simulink model "RobotSimulation"  (R2020b)
settings: Solver=ode45  StartTime=0.0  StopTime=2  MaxStep=1e-6  RelTol=1e-3%1e-10
model workspace (MAT data in the model file):
  Mchoice_Planned = Simulink.Parameter
  Mchoice_Planned.Value = 0
  Mchoice_Planned.DataType = 'auto'
  Mchoice_Planned.Dimensions = [1 1]
  robot = robotics.RigidBodyTree
  robot.TreeInternal = robotics.manip.internal.RigidBodyTree
  robot.TreeInternal.NumBodies = 4
  robot.TreeInternal.Base = robotics.manip.internal.RigidBody
  robot.TreeInternal.Base.Index = 0
  robot.TreeInternal.Base.NameInternal = 'base'
  robot.TreeInternal.Base.JointInternal = robotics.Joint
  robot.TreeInternal.Base.JointInternal.Type = 'fixed'
  robot.TreeInternal.Base.JointInternal.VelocityNumber = 0
  robot.TreeInternal.Base.JointInternal.PositionNumber = 0
  robot.TreeInternal.Base.JointInternal.MotionSubspace = [0; 0; 0; 0; 0; 0]
  robot.TreeInternal.Base.JointInternal.NameInternal = 'base_jnt'
  robot.TreeInternal.Base.ParentIndex = -1
  robot.TreeInternal.Base.ChildrenIndices = 1
  robot.TreeInternal.Base.MassInternal = 1
  robot.TreeInternal.Base.CenterOfMassInternal = [0 0 0]
  robot.TreeInternal.Base.InertiaInternal = [1  0  0; 0  1  0; 0  0  1]
  robot.TreeInternal.Base.SpatialInertia = [1  0  0  0  0  0; 0  1  0  0  0  0; 0  0  1  0  0  0; 0  0  0  1  0  0; 0  0  0  0  1  0; 0  0  0  0  0  1]
  robot.TreeInternal.Base.CollisionsInternal = robotics.manip.internal.CollisionSet
  robot.TreeInternal.Base.CollisionsInternal.MaxElements = 0
  robot.TreeInternal.Gravity = [0 0 0]
  robot.TreeInternal.Bodies{1} = robotics.manip.internal.RigidBody
  robot.TreeInternal.Bodies{1}.Index = 1
  robot.TreeInternal.Bodies{1}.NameInternal = 'body1'
  robot.TreeInternal.Bodies{1}.JointInternal = robotics.Joint
  robot.TreeInternal.Bodies{1}.JointInternal.Type = 'revolute'
  robot.TreeInternal.Bodies{1}.JointInternal.VelocityNumber = 1
  robot.TreeInternal.Bodies{1}.JointInternal.PositionNumber = 1
  robot.TreeInternal.Bodies{1}.JointInternal.MotionSubspace = [0; 0; 1; 0; 0; 0]
  robot.TreeInternal.Bodies{1}.JointInternal.InTree = 1
  robot.TreeInternal.Bodies{1}.JointInternal.NameInternal = 'jnt1'
  robot.TreeInternal.Bodies{1}.JointInternal.PositionLimitsInternal = [-3.14159265359 3.14159265359]
  robot.TreeInternal.Bodies{1}.JointInternal.JointAxisInternal = [0 0 1]
  robot.TreeInternal.Bodies{1}.ParentIndex = 0
  robot.TreeInternal.Bodies{1}.ChildrenIndices = [0 1]
  robot.TreeInternal.Bodies{1}.MassInternal = 1
  robot.TreeInternal.Bodies{1}.CenterOfMassInternal = [0 0 0]
  robot.TreeInternal.Bodies{1}.InertiaInternal = [1  0  0; 0  1  0; 0  0  1]
  robot.TreeInternal.Bodies{1}.SpatialInertia = [1  0  0  0  0  0; 0  1  0  0  0  0; 0  0  1  0  0  0; 0  0  0  1  0  0; 0  0  0  0  1  0; 0  0  0  0  0  1]
  robot.TreeInternal.Bodies{1}.CollisionsInternal = robotics.manip.internal.CollisionSet
  robot.TreeInternal.Bodies{1}.CollisionsInternal.MaxElements = 0
  robot.TreeInternal.Bodies{2} = robotics.manip.internal.RigidBody
  robot.TreeInternal.Bodies{2}.Index = 2
  robot.TreeInternal.Bodies{2}.NameInternal = 'body2'
  robot.TreeInternal.Bodies{2}.JointInternal = robotics.Joint
  robot.TreeInternal.Bodies{2}.JointInternal.Type = 'revolute'
  robot.TreeInternal.Bodies{2}.JointInternal.VelocityNumber = 1
  robot.TreeInternal.Bodies{2}.JointInternal.PositionNumber = 1
  robot.TreeInternal.Bodies{2}.JointInternal.MotionSubspace = [0; 0; 1; 0; 0; 0]
  robot.TreeInternal.Bodies{2}.JointInternal.InTree = 1
  robot.TreeInternal.Bodies{2}.JointInternal.JointToParentTransform = [1  0  0  0; 0  1  0  0; 0  0  1  0.2; 0  0  0  1]
  robot.TreeInternal.Bodies{2}.JointInternal.NameInternal = 'jnt2'
  robot.TreeInternal.Bodies{2}.JointInternal.PositionLimitsInternal = [-3.14159265359 3.14159265359]
  robot.TreeInternal.Bodies{2}.JointInternal.JointAxisInternal = [0 0 1]
  robot.TreeInternal.Bodies{2}.ParentIndex = 1
  robot.TreeInternal.Bodies{2}.ChildrenIndices = [0 0 1]
  robot.TreeInternal.Bodies{2}.MassInternal = 1
  robot.TreeInternal.Bodies{2}.CenterOfMassInternal = [0 0 0]
  robot.TreeInternal.Bodies{2}.InertiaInternal = [1  0  0; 0  1  0; 0  0  1]
  robot.TreeInternal.Bodies{2}.SpatialInertia = [1  0  0  0  0  0; 0  1  0  0  0  0; 0  0  1  0  0  0; 0  0  0  1  0  0; 0  0  0  0  1  0; 0  0  0  0  0  1]
  robot.TreeInternal.Bodies{2}.CollisionsInternal = robotics.manip.internal.CollisionSet
  robot.TreeInternal.Bodies{2}.CollisionsInternal.MaxElements = 0
  robot.TreeInternal.Bodies{3} = robotics.manip.internal.RigidBody
  robot.TreeInternal.Bodies{3}.Index = 3
  robot.TreeInternal.Bodies{3}.NameInternal = 'body3'
  robot.TreeInternal.Bodies{3}.JointInternal = robotics.Joint
  robot.TreeInternal.Bodies{3}.JointInternal.Type = 'prismatic'
  robot.TreeInternal.Bodies{3}.JointInternal.VelocityNumber = 1
  robot.TreeInternal.Bodies{3}.JointInternal.PositionNumber = 1
  robot.TreeInternal.Bodies{3}.JointInternal.MotionSubspace = [0; 0; 0; 0; 0; 1]
  robot.TreeInternal.Bodies{3}.JointInternal.InTree = 1
  robot.TreeInternal.Bodies{3}.JointInternal.JointToParentTransform = [1  0  0  0.1; 0  1  0  0; 0  0  1  0; 0  0  0  1]
  robot.TreeInternal.Bodies{3}.JointInternal.NameInternal = 'jnt3'
  robot.TreeInternal.Bodies{3}.JointInternal.PositionLimitsInternal = [-0.5 0.5]
  robot.TreeInternal.Bodies{3}.JointInternal.JointAxisInternal = [0 0 1]
  robot.TreeInternal.Bodies{3}.ParentIndex = 2
  robot.TreeInternal.Bodies{3}.ChildrenIndices = [0 0 0 1]
  robot.TreeInternal.Bodies{3}.MassInternal = 1
  robot.TreeInternal.Bodies{3}.CenterOfMassInternal = [0 0 0]
  robot.TreeInternal.Bodies{3}.InertiaInternal = [1  0  0; 0  1  0; 0  0  1]
  robot.TreeInternal.Bodies{3}.SpatialInertia = [1  0  0  0  0  0; 0  1  0  0  0  0; 0  0  1  0  0  0; 0  0  0  1  0  0; 0  0  0  0  1  0; 0  0  0  0  0  1]
  robot.TreeInternal.Bodies{3}.CollisionsInternal = robotics.manip.internal.CollisionSet
  robot.TreeInternal.Bodies{3}.CollisionsInternal.MaxElements = 0
  robot.TreeInternal.Bodies{4} = robotics.manip.internal.RigidBody
  robot.TreeInternal.Bodies{4}.Index = 4
  robot.TreeInternal.Bodies{4}.NameInternal = 'tool'
  robot.TreeInternal.Bodies{4}.JointInternal = robotics.Joint
  robot.TreeInternal.Bodies{4}.JointInternal.Type = 'fixed'
  robot.TreeInternal.Bodies{4}.JointInternal.VelocityNumber = 0
  robot.TreeInternal.Bodies{4}.JointInternal.PositionNumber = 0
  robot.TreeInternal.Bodies{4}.JointInternal.MotionSubspace = [0; 0; 0; 0; 0; 0]
  robot.TreeInternal.Bodies{4}.JointInternal.InTree = 1
  robot.TreeInternal.Bodies{4}.JointInternal.NameInternal = 'jnt4'
  robot.TreeInternal.Bodies{4}.ParentIndex = 3
  robot.TreeInternal.Bodies{4}.ChildrenIndices = [0 0 0]
  robot.TreeInternal.Bodies{4}.MassInternal = 1
  robot.TreeInternal.Bodies{4}.CenterOfMassInternal = [0 0 0]
  robot.TreeInternal.Bodies{4}.InertiaInternal = [1  0  0; 0  1  0; 0  0  1]
  robot.TreeInternal.Bodies{4}.SpatialInertia = [1  0  0  0  0  0; 0  1  0  0  0  0; 0  0  1  0  0  0; 0  0  0  1  0  0; 0  0  0  0  1  0; 0  0  0  0  0  1]
  robot.TreeInternal.Bodies{4}.CollisionsInternal = robotics.manip.internal.CollisionSet
  robot.TreeInternal.Bodies{4}.CollisionsInternal.MaxElements = 0
  robot.TreeInternal.NumNonFixedBodies = 3
  robot.TreeInternal.PositionNumber = 3
  robot.TreeInternal.VelocityNumber = 3
  robot.TreeInternal.PositionDoFMap = [1  1; 2  2; 3  3; 0  -1]
  robot.TreeInternal.VelocityDoFMap = [1  1; 2  2; 3  3; 0  -1]
  robot.TreeInternal.MaxNumBodies = 4
  robot.TreeInternal.MaxNameLength = 200
  robot.TreeInternal.MaxJointPositionNumber = 7
  robot.TreeInternal.VisualizationInfo = robotics.manip.internal.VisualizationInfo
  robot.TreeInternal.VisualizationInfo.ShowTag = 'DO_NOT_EDIT_qoTUB'
  robot.TreeInternal.DataFormatInternal = 'struct'
settings Model: OrderedModelArguments=off  Creator=alons  LastModifiedBy=alons
settings SolverCC: ConsecutiveZCsStepRelTol=eps%10*128*eps

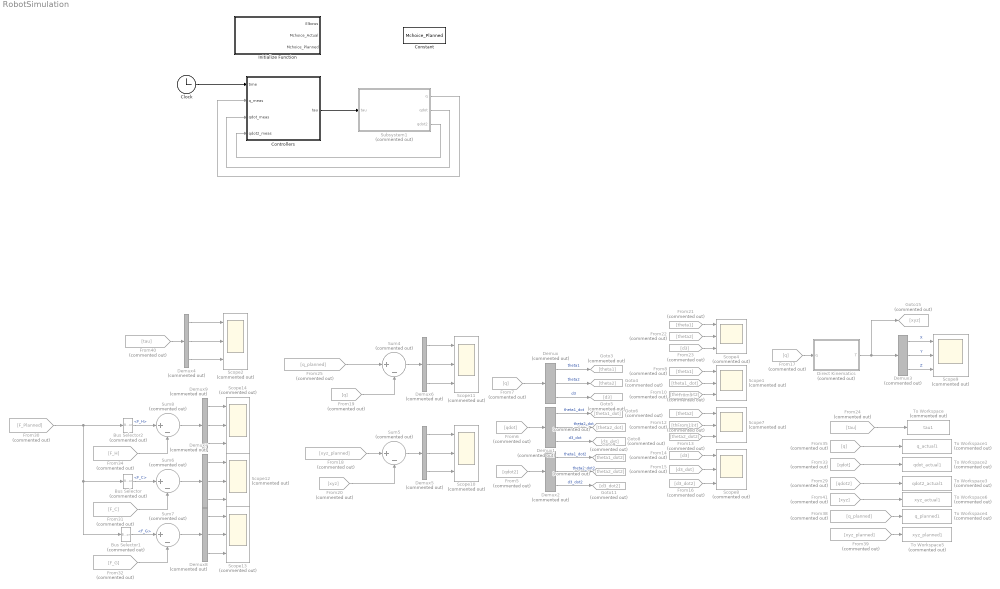
== system RobotSimulation ==
  Bus Selector : BusSelector  Commented=on  OutputSignals=F_C
  Bus Selector1 : BusSelector  Commented=on  OutputSignals=F_G
  Bus Selector2 : BusSelector  Commented=on  OutputSignals=F_H
  Clock : Clock
  Constant : Constant  Value=Mchoice_Planned
  Controllers : Subsystem  TreatAsAtomicUnit=on
      mask Display: disp('Controller')
  Demux{,1..9} (10 alike) : Demux  Commented=on  Outputs=3
  Direct Kinematics : MATLAB Function  Commented=on  TreatAsAtomicUnit=on
  From10 : From  Commented=on  GotoTag=theta1_dot2
  From11 : From  Commented=on  GotoTag=theta2
  From12 : From  Commented=on  GotoTag=theta2_dot
  From13 : From  Commented=on  GotoTag=theta2_dot2
  From14 : From  Commented=on  GotoTag=d3
  From15 : From  Commented=on  GotoTag=d3_dot
  From16 : From  Commented=on  GotoTag=d3_dot2
  From{7,17,19,35} (4 alike) : From  Commented=on  GotoTag=q
  From18 : From  Commented=on  GotoTag=xyz_planned
  From20 : From  Commented=on  GotoTag=xyz
  From21 : From  Commented=on  GotoTag=theta1
  From22 : From  Commented=on  GotoTag=theta2
  From23 : From  Commented=on  GotoTag=d3
  From24 : From  Commented=on  GotoTag=tau
  From25 : From  Commented=on  GotoTag=q_planned
  From29 : From  Commented=on  GotoTag=qdot2
  From30 : From  Commented=on  GotoTag=F_Planned
  From31 : From  Commented=on  GotoTag=F_C
  From32 : From  Commented=on  GotoTag=F_G
  From33 : From  Commented=on  GotoTag=qdot
  From34 : From  Commented=on  GotoTag=F_H
  From38 : From  Commented=on  GotoTag=q_planned
  From39 : From  Commented=on  GotoTag=xyz_planned
  From40 : From  Commented=on  GotoTag=tau
  From41 : From  Commented=on  GotoTag=xyz
  From5 : From  Commented=on  GotoTag=qdot2
  From6 : From  Commented=on  GotoTag=qdot
  From8 : From  Commented=on  GotoTag=theta1
  From9 : From  Commented=on  GotoTag=theta1_dot
  Goto10 : Goto  Commented=on  GotoTag=theta2_dot2
  Goto11 : Goto  Commented=on  GotoTag=d3_dot2
  Goto15 : Goto  Commented=on  GotoTag=xyz
  Goto3 : Goto  Commented=on  GotoTag=theta1
  Goto4 : Goto  Commented=on  GotoTag=theta2
  Goto5 : Goto  Commented=on  GotoTag=d3
  Goto6 : Goto  Commented=on  GotoTag=theta1_dot
  Goto7 : Goto  Commented=on  GotoTag=theta2_dot
  Goto8 : Goto  Commented=on  GotoTag=d3_dot
  Goto9 : Goto  Commented=on  GotoTag=theta1_dot2
  Initialize Function : Subsystem  TreatAsAtomicUnit=on
  Scope{1..2,4,7..14} (11 alike) : Scope  Commented=on  NumInputPorts=3
  Subsystem1 : Subsystem  Commented=on
      mask Display: disp('Plant')
  Sum{4..8} (5 alike) : Sum  Commented=on  Inputs=|+-
  To Workspace : ToWorkspace  Commented=on  VariableName=tau1  SaveFormat=Timeseries  SampleTime=-1
  To Workspace1 : ToWorkspace  Commented=on  VariableName=q_actual1  SaveFormat=Timeseries  SampleTime=-1
  To Workspace2 : ToWorkspace  Commented=on  VariableName=qdot_actual1  SaveFormat=Timeseries  SampleTime=-1
  To Workspace3 : ToWorkspace  Commented=on  VariableName=qdot2_actual1  SaveFormat=Timeseries  SampleTime=-1
  To Workspace4 : ToWorkspace  Commented=on  VariableName=q_planned1  SaveFormat=Timeseries  SampleTime=-1
  To Workspace5 : ToWorkspace  Commented=on  VariableName=xyz_planned1  SaveFormat=Timeseries  SampleTime=-1
  To Workspace6 : ToWorkspace  Commented=on  VariableName=xyz_actual1  SaveFormat=Timeseries  SampleTime=-1
  wires:
  Demux3/3 -> Scope9/3  "Z"
  From17/1 -> Direct Kinematics/1(q)
  From7/1 -> Demux/1
  Demux9/2 -> Scope14/2
  From41/1 -> To Workspace6/1
  Demux4/3 -> Scope2/3
  Demux8/1 -> Scope13/1
  Demux4/1 -> Scope2/1
  Demux3/1 -> Scope9/1  "X"
  From20/1 -> Sum5/2
  From13/1 -> Scope7/3
  From18/1 -> Sum5/1
  From22/1 -> Scope4/2
  Demux/2 -> Goto4/1  "theta2"
  From23/1 -> Scope4/3
  Demux5/1 -> Scope10/1
  Demux1/2 -> Goto7/1  "theta2_dot"
  From21/1 -> Scope4/1
  From6/1 -> Demux1/1
  From8/1 -> Scope1/1
  Demux2/1 -> Goto9/1  "theta1_dot2"
  Demux1/3 -> Goto8/1  "d3_dot"
  From11/1 -> Scope7/1
  From32/1 -> Sum7/2
  Direct Kinematics/1(T) -> Goto15/1, Demux3/1
  Demux7/3 -> Scope12/3
  Bus Selector1/1 -> Sum7/1  "<F_G>"
  From19/1 -> Sum4/2
  Sum7/1 -> Demux8/1
  From14/1 -> Scope8/1
  Demux8/2 -> Scope13/2
  From31/1 -> Sum6/2
  Demux8/3 -> Scope13/3
  Demux3/2 -> Scope9/2  "Y"
  From9/1 -> Scope1/2
  Demux9/3 -> Scope14/3
  Demux2/3 -> Goto11/1  "d3_dot2"
  From34/1 -> Sum8/2
  Sum6/1 -> Demux7/1
  Demux4/2 -> Scope2/2
  From15/1 -> Scope8/2
  Sum8/1 -> Demux9/1
  Demux6/3 -> Scope11/3
  Sum5/1 -> Demux5/1
  Bus Selector2/1 -> Sum8/1  "<F_H>"
  From30/1 -> Bus Selector1/1, Bus Selector/1, Bus Selector2/1
  Demux/1 -> Goto3/1  "theta1"
  Demux2/2 -> Goto10/1  "theta2_dot2"
  From12/1 -> Scope7/2
  From24/1 -> To Workspace/1
  Sum4/1 -> Demux6/1
  Demux5/3 -> Scope10/3
  From29/1 -> To Workspace3/1
  Demux9/1 -> Scope14/1
  Demux7/2 -> Scope12/2
  Demux5/2 -> Scope10/2
  From16/1 -> Scope8/3
  Demux7/1 -> Scope12/1
  From39/1 -> To Workspace5/1
  From25/1 -> Sum4/1
  Demux6/2 -> Scope11/2
  Demux/3 -> Goto5/1  "d3"
  From35/1 -> To Workspace1/1
  Demux1/1 -> Goto6/1  "theta1_dot"
  From38/1 -> To Workspace4/1
  Bus Selector/1 -> Sum6/1  "<F_C>"
  Demux6/1 -> Scope11/1
  From10/1 -> Scope1/3
  From33/1 -> To Workspace2/1
  From5/1 -> Demux2/1
  From40/1 -> Demux4/1
  Clock/1 -> Controllers/1(time)
  Controllers/1(tau) -> Subsystem1/1(tau)
  Subsystem1/1(q) -> Controllers/2(q_meas)
  Subsystem1/2(qdot) -> Controllers/3(qdot_meas)
  Subsystem1/3(qdot2) -> Controllers/4(qdot2_meas)

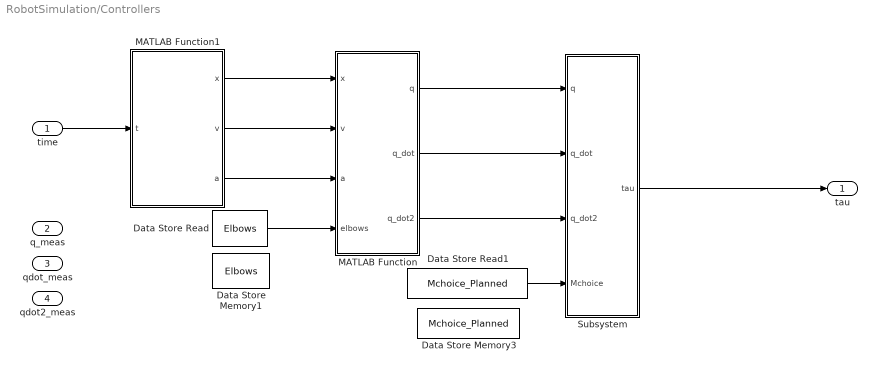
== system RobotSimulation/Controllers ==
  time : Inport
  q_meas : Inport  Port=2
  qdot_meas : Inport  Port=3
  qdot2_meas : Inport  Port=4
  Data Store Memory1 : DataStoreMemory  DataStoreName=Elbows  ReadBeforeWriteMsg=warning  WriteAfterWriteMsg=warning  WriteAfterReadMsg=warning  ShowAdditionalParam=off
  Data Store Memory3 : DataStoreMemory  DataStoreName=Mchoice_Planned  ReadBeforeWriteMsg=warning  WriteAfterWriteMsg=warning  WriteAfterReadMsg=warning  ShowAdditionalParam=off
  Data Store Read : DataStoreRead  DataStoreName=Elbows  DataStoreElements=Elbows
  Data Store Read1 : DataStoreRead  DataStoreName=Mchoice_Planned  DataStoreElements=Mchoice_Planned
  MATLAB Function : MATLAB Function  TreatAsAtomicUnit=on
  MATLAB Function1 : MATLAB Function  TreatAsAtomicUnit=on
  Subsystem : Subsystem
  tau : Outport
  wires:
  MATLAB Function1/3(a) -> MATLAB Function/3(a)
  Data Store Read/1 -> MATLAB Function/4(elbows)
  Data Store Read1/1 -> Subsystem/4(Mchoice)
  MATLAB Function/2(q_dot) -> Subsystem/2(q_dot)
  MATLAB Function1/1(x) -> MATLAB Function/1(x)
  MATLAB Function/3(q_dot2) -> Subsystem/3(q_dot2)
  MATLAB Function/1(q) -> Subsystem/1(q)
  MATLAB Function1/2(v) -> MATLAB Function/2(v)
  time/1 -> MATLAB Function1/1(t)
  Subsystem/1(tau) -> tau/1

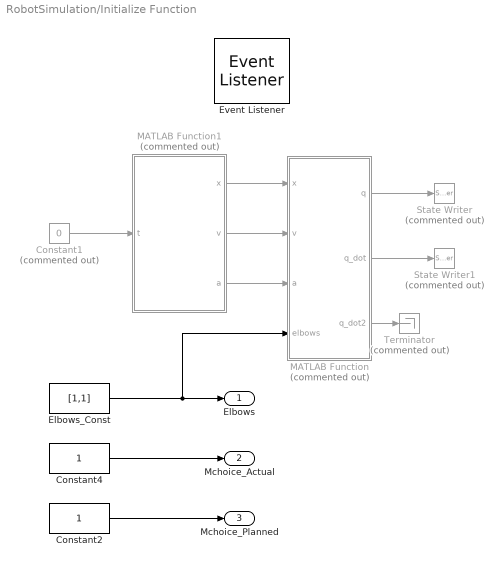
== system RobotSimulation/Initialize Function ==
  Constant1 : Constant  Commented=on  Value=0
  Constant2 : Constant
  Constant4 : Constant
  Elbows_Const : Constant  Value=[1,1]
  Event Listener : EventListener  DisableCoverage=on  EventName=reset
  MATLAB Function : MATLAB Function  Commented=on  TreatAsAtomicUnit=on
  MATLAB Function1 : MATLAB Function  Commented=on  TreatAsAtomicUnit=on
  State Writer : StateWriter  Commented=on  StateOwnerBlock=../../Subsystem1/Int_2q
  State Writer1 : StateWriter  Commented=on  StateOwnerBlock=../../Subsystem1/Int_2qdot
  Terminator : Terminator  Commented=on
  Elbows : Outport
  Mchoice_Actual : Outport  Port=2
  Mchoice_Planned : Outport  Port=3
  wires:
  Constant1/1 -> MATLAB Function1/1(t)
  MATLAB Function1/1(x) -> MATLAB Function/1(x)
  MATLAB Function1/2(v) -> MATLAB Function/2(v)
  MATLAB Function1/3(a) -> MATLAB Function/3(a)
  Elbows_Const/1 -> Elbows/1, MATLAB Function/4(elbows)
  MATLAB Function/1(q) -> State Writer/1
  MATLAB Function/2(q_dot) -> State Writer1/1
  MATLAB Function/3(q_dot2) -> Terminator/1
  Constant4/1 -> Mchoice_Actual/1
  Constant2/1 -> Mchoice_Planned/1

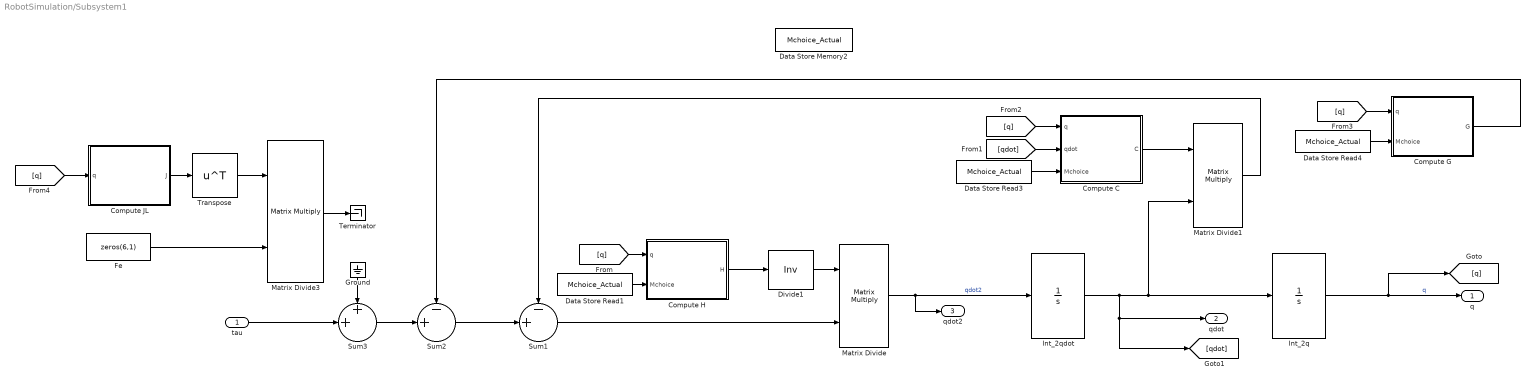
== system RobotSimulation/Subsystem1 ==
  tau : Inport
  Compute C : MATLAB Function  TreatAsAtomicUnit=on
  Compute G : MATLAB Function  TreatAsAtomicUnit=on
  Compute H : MATLAB Function  TreatAsAtomicUnit=on
  Compute JL : MATLAB Function  TreatAsAtomicUnit=on
  Data Store Memory2 : DataStoreMemory  DataStoreName=Mchoice_Actual  ReadBeforeWriteMsg=warning  WriteAfterWriteMsg=warning  WriteAfterReadMsg=warning  ShowAdditionalParam=off
  Data Store Read1 : DataStoreRead  DataStoreName=Mchoice_Actual  DataStoreElements=Mchoice_Actual
  Data Store Read3 : DataStoreRead  DataStoreName=Mchoice_Actual  DataStoreElements=Mchoice_Actual
  Data Store Read4 : DataStoreRead  DataStoreName=Mchoice_Actual  DataStoreElements=Mchoice_Actual
  Divide1 : Product  Inputs=/  Multiplication=Matrix(*)
  Fe : Constant  Value=zeros(6,1)
  Ground : Ground
  Int_2q : Integrator  InitialCondition=[0,0,0]'
  Int_2qdot : Integrator  InitialCondition=[0,0,0]'
  Matrix Divide : Product  Inputs=**  Multiplication=Matrix(*)
  Matrix Divide1 : Product  Inputs=**  Multiplication=Matrix(*)
  Matrix Divide3 : Product  Inputs=**  Multiplication=Matrix(*)
  Sum1 : Sum  Inputs=-+|
  Sum2 : Sum  Inputs=-+|
  Sum3 : Sum  Inputs=++|
  Terminator : Terminator
  Transpose : Math  Operator=transpose  SaturateOnIntegerOverflow=on
  q : Outport
  qdot : Outport  Port=2
  qdot2 : Outport  Port=3
  wires:
  Sum1/1 -> Matrix Divide/2
  Matrix Divide3/1 -> Terminator/1
  [q] -> Compute C/1(q)
  [qdot] -> Compute C/2(qdot)
  Int_2q/1 -> q/1, [q]  "q"
  Data Store Read4/1 -> Compute G/2(Mchoice)
  Compute C/1(C) -> Matrix Divide1/1
  Ground/1 -> Sum3/1
  Data Store Read1/1 -> Compute H/2(Mchoice)
  Compute G/1(G) -> Sum2/1
  Divide1/1 -> Matrix Divide/1
  Fe/1 -> Matrix Divide3/2
  Int_2qdot/1 -> Int_2q/1, Matrix Divide1/2, [qdot], qdot/1
  Data Store Read3/1 -> Compute C/3(Mchoice)
  Compute H/1(H) -> Divide1/1
  Sum2/1 -> Sum1/2
  Matrix Divide/1 -> qdot2/1, Int_2qdot/1  "qdot2"
  [q] -> Compute H/1(q)
  Transpose/1 -> Matrix Divide3/1
  Compute JL/1(J) -> Transpose/1
  Sum3/1 -> Sum2/2
  [q] -> Compute JL/1(q)
  [q] -> Compute G/1(q)
  tau/1 -> Sum3/2
  Matrix Divide1/1 -> Sum1/1

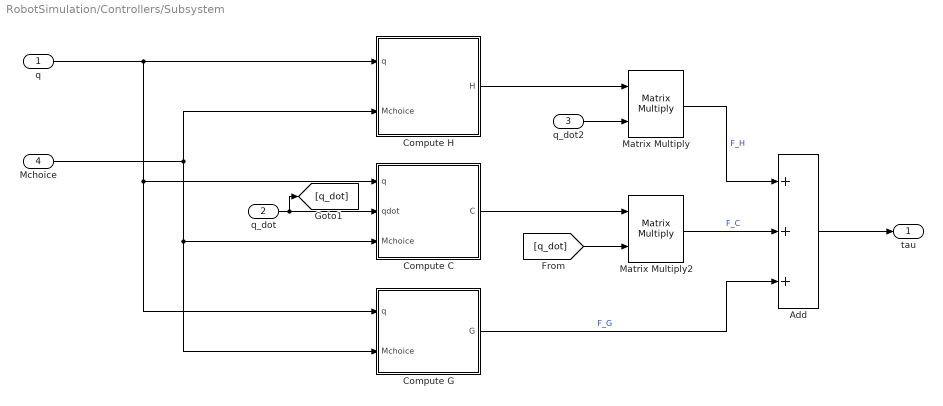
== system RobotSimulation/Controllers/Subsystem ==
  q : Inport
  q_dot : Inport  Port=2
  q_dot2 : Inport  Port=3
  Mchoice : Inport  Port=4
  Add : Sum  Inputs=+++
  Compute C : MATLAB Function  TreatAsAtomicUnit=on
  Compute G : MATLAB Function  TreatAsAtomicUnit=on
  Compute H : MATLAB Function  TreatAsAtomicUnit=on
  Matrix Multiply : Product  Multiplication=Matrix(*)
  Matrix Multiply2 : Product  Multiplication=Matrix(*)
  tau : Outport
  wires:
  Compute H/1(H) -> Matrix Multiply/1
  Compute C/1(C) -> Matrix Multiply2/1
  q/1 -> Compute H/1(q), Compute G/1(q), Compute C/1(q)
  q_dot/1 -> [q_dot], Compute C/2(qdot)
  q_dot2/1 -> Matrix Multiply/2
  [q_dot] -> Matrix Multiply2/2
  Matrix Multiply/1 -> Add/1  "F_H"
  Add/1 -> tau/1
  Matrix Multiply2/1 -> Add/2  "F_C"
  Compute G/1(G) -> Add/3  "F_G"
  Mchoice/1 -> Compute H/2(Mchoice), Compute G/2(Mchoice), Compute C/3(Mchoice)

== matlab function RobotSimulation/Controllers/Subsystem/Compute G ==
  data: q input; G output; Mchoice input
function G = ComputeG(q,Mchoice)
f_GdynM1=@(in1)[0.0;sin(in1(2,:)).*(in1(3,:).*1.0e+1-pi.*4.3875e-2+in1(3,:).*pi.*(3.51e+2./4.0e+2)).*(-4.905e-1);cos(in1(2,:)).*(pi.*4.3875e-2+1.0./2.0).*(9.81e+2./1.0e+2)];
f_GdynM2=@(in1)[0.0;sin(in1(2,:)).*(in1(3,:).*1.2e+1-pi.*4.3875e-2+in1(3,:).*pi.*(3.51e+2./4.0e+2)).*(-4.905e-1);cos(in1(2,:)).*(pi.*4.3875e-2+3.0./5.0).*(9.81e+2./1.0e+2)];
if Mchoice==1
    G=f_GdynM1(q);
else %==2
    G=f_GdynM2(q);
end
end

== matlab function RobotSimulation/Controllers/Subsystem/Compute H ==
  data: q input; H output; Mchoice input
function H = ComputeH(q,Mchoice)
f_HdynM1=@(in1)reshape([pi.*5.85e-4+(in1(3,:).^2.*sin(in1(2,:)).^2)./2.0+pi.*sin(in1(2,:)).^2.*1.4625e-4-in1(3,:).*pi.*sin(in1(2,:)).^2.*4.3875e-3+in1(3,:).^2.*pi.*sin(in1(2,:)).^2.*4.3875e-2+1.0./2.0e+2,cos(in1(2,:)).*(in1(3,:).*1.0e+1-pi.*4.3875e-2+in1(3,:).*pi.*(3.51e+2./4.0e+2)).*(-1.0./2.0e+2),sin(in1(2,:)).*(pi.*4.3875e-2+1.0./2.0).*(-1.0./1.0e+1),cos(in1(2,:)).*(in1(3,:).*1.0e+1-pi.*4.3875e-2+in1(3,:).*pi.*(3.51e+2./4.0e+2)).*(-1.0./2.0e+2),pi.*3.65625e-5+in1(3,:).^2./2.0+pi.*(in1(3,:)-1.0./2.0e+1).^2.*4.3875e-2,0.0,sin(in1(2,:)).*(pi.*4.3875e-2+1.0./2.0).*(-1.0./1.0e+1),0.0,pi.*4.3875e-2+1.0./2.0],[3,3]);
f_HdynM2=@(in1)reshape([pi.*5.85e-4+in1(3,:).^2.*sin(in1(2,:)).^2.*(3.0./5.0)+pi.*sin(in1(2,:)).^2.*1.4625e-4-in1(3,:).*pi.*sin(in1(2,:)).^2.*4.3875e-3+in1(3,:).^2.*pi.*sin(in1(2,:)).^2.*4.3875e-2+3.0./5.0e+2,cos(in1(2,:)).*(in1(3,:).*1.2e+1-pi.*4.3875e-2+in1(3,:).*pi.*(3.51e+2./4.0e+2)).*(-1.0./2.0e+2),sin(in1(2,:)).*(pi.*4.3875e-2+3.0./5.0).*(-1.0./1.0e+1),cos(in1(2,:)).*(in1(3,:).*1.2e+1-pi.*4.3875e-2+in1(3,:).*pi.*(3.51e+2./4.0e+2)).*(-1.0./2.0e+2),pi.*3.65625e-5+in1(3,:).^2.*(3.0./5.0)+pi.*(in1(3,:)-1.0./2.0e+1).^2.*4.3875e-2,0.0,sin(in1(2,:)).*(pi.*4.3875e-2+3.0./5.0).*(-1.0./1.0e+1),0.0,pi.*4.3875e-2+3.0./5.0],[3,3]);
if Mchoice==1
    H=f_HdynM1(q);
else %==2
    H=f_HdynM2(q);
end

== matlab function RobotSimulation/Subsystem1/Compute C ==
  data: q input; C output; qdot input; Mchoice input
function C = ComputeC(q,qdot,Mchoice)
f_CdynM1=@(in1)reshape([in1(6,:).*((in1(3,:).*sin(in1(2,:)).^2)./2.0-pi.*sin(in1(2,:)).^2.*2.19375e-3+in1(3,:).*pi.*sin(in1(2,:)).^2.*4.3875e-2)+in1(5,:).*((in1(3,:).^2.*sin(in1(2,:).*2.0))./4.0+pi.*sin(in1(2,:).*2.0).*7.3125e-5-in1(3,:).*pi.*sin(in1(2,:).*2.0).*2.19375e-3+in1(3,:).^2.*pi.*sin(in1(2,:).*2.0).*2.19375e-2),in1(4,:).*sin(in1(2,:).*2.0).*(pi.*1.755e-1-in1(3,:).*pi.*5.265+in1(3,:).^2.*pi.*5.265e+1+in1(3,:).^2.*6.0e+2).*(-4.166666666666667e-4),in1(4,:).*sin(in1(2,:)).^2.*(in1(3,:).*1.0e+1-pi.*4.3875e-2+in1(3,:).*pi.*(3.51e+2./4.0e+2)).*(-1.0./2.0e+1),in1(4,:).*((in1(3,:).^2.*sin(in1(2,:).*2.0))./4.0+pi.*sin(in1(2,:).*2.0).*7.3125e-5-in1(3,:).*pi.*sin(in1(2,:).*2.0).*2.19375e-3+in1(3,:).^2.*pi.*sin(in1(2,:).*2.0).*2.19375e-2)-in1(6,:).*((cos(in1(2,:)).*(pi.*(3.51e+2./4.0e+2)+1.0e+1))./4.0e+2+(cos(in1(2,:)).*(pi.*4.3875e-2+1.0./2.0))./2.0e+1)+(in1(5,:).*sin(in1(2,:)).*(in1(3,:).*1.0e+1-pi.*4.3875e-2+in1(3,:).*pi.*(3.51e+2./4.0e+2)))./2.0e+2,in1(6,:).*(in1(3,:)./2.0+pi.*(in1(3,:).*2.0-1.0./1.0e+1).*2.19375e-2),in1(5,:).*(in1(3,:).*1.0e+1-pi.*4.3875e-2+in1(3,:).*pi.*(3.51e+2./4.0e+2)).*(-1.0./2.0e+1),-in1(4,:).*(pi.*(cos(in1(2,:)).^2-1.0).*(-2.19375e-3)+(in1(3,:).*(cos(in1(2,:)).^2-1.0))./2.0+in1(3,:).*pi.*(cos(in1(2,:)).^2-1.0).*4.3875e-2)-in1(5,:).*((cos(in1(2,:)).*(pi.*(3.51e+2./4.0e+2)+1.0e+1))./4.0e+2+(cos(in1(2,:)).*(pi.*4.3875e-2+1.0./2.0))./2.0e+1),(in1(5,:).*(in1(3,:).*1.0e+1-pi.*4.3875e-2+in1(3,:).*pi.*(3.51e+2./4.0e+2)))./2.0e+1,0.0],[3,3]);
f_CdynM2=@(in1)reshape([in1(6,:).*(in1(3,:).*sin(in1(2,:)).^2.*(3.0./5.0)-pi.*sin(in1(2,:)).^2.*2.19375e-3+in1(3,:).*pi.*sin(in1(2,:)).^2.*4.3875e-2)+in1(5,:).*(in1(3,:).^2.*sin(in1(2,:).*2.0).*(3.0./1.0e+1)+pi.*sin(in1(2,:).*2.0).*7.3125e-5-in1(3,:).*pi.*sin(in1(2,:).*2.0).*2.19375e-3+in1(3,:).^2.*pi.*sin(in1(2,:).*2.0).*2.19375e-2),in1(4,:).*sin(in1(2,:).*2.0).*(pi.*1.755e-1-in1(3,:).*pi.*5.265+in1(3,:).^2.*pi.*5.265e+1+in1(3,:).^2.*7.2e+2).*(-4.166666666666667e-4),in1(4,:).*sin(in1(2,:)).^2.*(in1(3,:).*1.2e+1-pi.*4.3875e-2+in1(3,:).*pi.*(3.51e+2./4.0e+2)).*(-1.0./2.0e+1),in1(4,:).*(in1(3,:).^2.*sin(in1(2,:).*2.0).*(3.0./1.0e+1)+pi.*sin(in1(2,:).*2.0).*7.3125e-5-in1(3,:).*pi.*sin(in1(2,:).*2.0).*2.19375e-3+in1(3,:).^2.*pi.*sin(in1(2,:).*2.0).*2.19375e-2)-in1(6,:).*((cos(in1(2,:)).*(pi.*(3.51e+2./4.0e+2)+1.2e+1))./4.0e+2+(cos(in1(2,:)).*(pi.*4.3875e-2+3.0./5.0))./2.0e+1)+(in1(5,:).*sin(in1(2,:)).*(in1(3,:).*1.2e+1-pi.*4.3875e-2+in1(3,:).*pi.*(3.51e+2./4.0e+2)))./2.0e+2,in1(6,:).*(in1(3,:).*(3.0./5.0)+pi.*(in1(3,:).*2.0-1.0./1.0e+1).*2.19375e-2),in1(5,:).*(in1(3,:).*1.2e+1-pi.*4.3875e-2+in1(3,:).*pi.*(3.51e+2./4.0e+2)).*(-1.0./2.0e+1),-in1(4,:).*(pi.*(cos(in1(2,:)).^2-1.0).*(-2.19375e-3)+in1(3,:).*(cos(in1(2,:)).^2-1.0).*(3.0./5.0)+in1(3,:).*pi.*(cos(in1(2,:)).^2-1.0).*4.3875e-2)-in1(5,:).*((cos(in1(2,:)).*(pi.*(3.51e+2./4.0e+2)+1.2e+1))./4.0e+2+(cos(in1(2,:)).*(pi.*4.3875e-2+3.0./5.0))./2.0e+1),(in1(5,:).*(in1(3,:).*1.2e+1-pi.*4.3875e-2+in1(3,:).*pi.*(3.51e+2./4.0e+2)))./2.0e+1,0.0],[3,3]);
if Mchoice==1
    C=f_CdynM1([q;qdot]);
else %==2
    C=f_CdynM2([q;qdot]);
end
end

== matlab function RobotSimulation/Subsystem1/Compute H ==
  data: q input; H output; Mchoice input
function H = ComputeH(q,Mchoice)
f_HdynM1=@(in1)reshape([pi.*5.85e-4+(in1(3,:).^2.*sin(in1(2,:)).^2)./2.0+pi.*sin(in1(2,:)).^2.*1.4625e-4-in1(3,:).*pi.*sin(in1(2,:)).^2.*4.3875e-3+in1(3,:).^2.*pi.*sin(in1(2,:)).^2.*4.3875e-2+1.0./2.0e+2,cos(in1(2,:)).*(in1(3,:).*1.0e+1-pi.*4.3875e-2+in1(3,:).*pi.*(3.51e+2./4.0e+2)).*(-1.0./2.0e+2),sin(in1(2,:)).*(pi.*4.3875e-2+1.0./2.0).*(-1.0./1.0e+1),cos(in1(2,:)).*(in1(3,:).*1.0e+1-pi.*4.3875e-2+in1(3,:).*pi.*(3.51e+2./4.0e+2)).*(-1.0./2.0e+2),pi.*3.65625e-5+in1(3,:).^2./2.0+pi.*(in1(3,:)-1.0./2.0e+1).^2.*4.3875e-2,0.0,sin(in1(2,:)).*(pi.*4.3875e-2+1.0./2.0).*(-1.0./1.0e+1),0.0,pi.*4.3875e-2+1.0./2.0],[3,3]);
f_HdynM2=@(in1)reshape([pi.*5.85e-4+in1(3,:).^2.*sin(in1(2,:)).^2.*(3.0./5.0)+pi.*sin(in1(2,:)).^2.*1.4625e-4-in1(3,:).*pi.*sin(in1(2,:)).^2.*4.3875e-3+in1(3,:).^2.*pi.*sin(in1(2,:)).^2.*4.3875e-2+3.0./5.0e+2,cos(in1(2,:)).*(in1(3,:).*1.2e+1-pi.*4.3875e-2+in1(3,:).*pi.*(3.51e+2./4.0e+2)).*(-1.0./2.0e+2),sin(in1(2,:)).*(pi.*4.3875e-2+3.0./5.0).*(-1.0./1.0e+1),cos(in1(2,:)).*(in1(3,:).*1.2e+1-pi.*4.3875e-2+in1(3,:).*pi.*(3.51e+2./4.0e+2)).*(-1.0./2.0e+2),pi.*3.65625e-5+in1(3,:).^2.*(3.0./5.0)+pi.*(in1(3,:)-1.0./2.0e+1).^2.*4.3875e-2,0.0,sin(in1(2,:)).*(pi.*4.3875e-2+3.0./5.0).*(-1.0./1.0e+1),0.0,pi.*4.3875e-2+3.0./5.0],[3,3]);
if Mchoice==1
    H=f_HdynM1(q);
else %==2
    H=f_HdynM2(q);
end

== matlab function RobotSimulation/Subsystem1/Compute G ==
  data: q input; G output; Mchoice input
function G = ComputeG(q,Mchoice)
f_GdynM1=@(in1)[0.0;sin(in1(2,:)).*(in1(3,:).*1.0e+1-pi.*4.3875e-2+in1(3,:).*pi.*(3.51e+2./4.0e+2)).*(-4.905e-1);cos(in1(2,:)).*(pi.*4.3875e-2+1.0./2.0).*(9.81e+2./1.0e+2)];
f_GdynM2=@(in1)[0.0;sin(in1(2,:)).*(in1(3,:).*1.2e+1-pi.*4.3875e-2+in1(3,:).*pi.*(3.51e+2./4.0e+2)).*(-4.905e-1);cos(in1(2,:)).*(pi.*4.3875e-2+3.0./5.0).*(9.81e+2./1.0e+2)];
if Mchoice==1
    G=f_GdynM1(q);
else %==2
    G=f_GdynM2(q);
end
end

== matlab function RobotSimulation/Subsystem1/Compute JL ==
  data: q input; J output
function J = ComputeJL(q)
f_JL=@(in1)reshape([sin(in1(1,:)).*(-1.0./1.0e+1)+in1(3,:).*cos(in1(1,:)).*sin(in1(2,:)),cos(in1(1,:))./1.0e+1+in1(3,:).*sin(in1(1,:)).*sin(in1(2,:)),0.0,in1(3,:).*cos(in1(2,:)).*sin(in1(1,:)),-in1(3,:).*cos(in1(1,:)).*cos(in1(2,:)),-in1(3,:).*sin(in1(2,:)),sin(in1(1,:)).*sin(in1(2,:)),-cos(in1(1,:)).*sin(in1(2,:)),cos(in1(2,:))],[3,3]);
f_JA=@(in1)reshape([0.0,0.0,1.0,cos(in1(1,:)),sin(in1(1,:)),0.0,0.0,0.0,0.0],[3,3]);
JL=f_JL(q);
JA=f_JA(q);
J=[JL;JA];
end

== matlab function RobotSimulation/Controllers/MATLAB Function ==
  data: x input; v input; a input; q output; elbows input; q_dot output; q_dot2 output
function [q,q_dot,q_dot2] = xyz2q(x,v,a,elbows)
q=inverse_kin(x,elbows);

JL=CalcJL(q);
q_dot=linsolve((JL),v);

JL_dot=CalcJLdot(q,q_dot);
q_dot2=linsolve(JL,a-JL_dot*q_dot);
end

function q=inverse_kin(x,elbows)
H=0.2;
L=0.1;

t2_elbow=elbows(1);
d3_elbow=elbows(2);
q=zeros(3,size(x,2));
for i=1:size(x,2)
    %Parse
    Px=x(1,i);
    Py=x(2,i);
    Pz=x(3,i);
    %Compute d3
    d3=d3_elbow*sqrt(Px^2+Py^2+(Pz-H)^2-L^2);
    %compute theta2
    c2=(Pz-H)/(d3+eps); %<------------Added eps
    s2=t2_elbow*sqrt(1-c2^2);
    t2=atan2(s2,c2);
    %compute theta1
    a=d3*s2;
    b=L;
    c=-Py;
    d=Px;
    t1=atan2(a*d-b*c,a*c+b*d);
    %create joint vector
    q(:,i)=[t1,t2,d3]';
end
end

function JL=CalcJL(q)
f_JL=@(in1)reshape([sin(in1(1,:)).*(-1.0./1.0e+1)+in1(3,:).*cos(in1(1,:)).*sin(in1(2,:)),cos(in1(1,:))./1.0e+1+in1(3,:).*sin(in1(1,:)).*sin(in1(2,:)),0.0,in1(3,:).*cos(in1(2,:)).*sin(in1(1,:)),-in1(3,:).*cos(in1(1,:)).*cos(in1(2,:)),-in1(3,:).*sin(in1(2,:)),sin(in1(1,:)).*sin(in1(2,:)),-cos(in1(1,:)).*sin(in1(2,:)),cos(in1(2,:))],[3,3]);
JL=f_JL(q);
end

function JLdot=CalcJLdot(q,qdot)
f_JLdot=@(in1)reshape([-in1(4,:).*(cos(in1(1,:))./1.0e+1+in1(3,:).*sin(in1(1,:)).*sin(in1(2,:)))+in1(6,:).*cos(in1(1,:)).*sin(in1(2,:))+in1(3,:).*in1(5,:).*cos(in1(1,:)).*cos(in1(2,:)),-in1(4,:).*(sin(in1(1,:))./1.0e+1-in1(3,:).*cos(in1(1,:)).*sin(in1(2,:)))+in1(6,:).*sin(in1(1,:)).*sin(in1(2,:))+in1(3,:).*in1(5,:).*cos(in1(2,:)).*sin(in1(1,:)),0.0,in1(6,:).*cos(in1(2,:)).*sin(in1(1,:))-in1(3,:).*in1(5,:).*sin(in1(1,:)).*sin(in1(2,:))+in1(3,:).*in1(4,:).*cos(in1(1,:)).*cos(in1(2,:)),-in1(6,:).*cos(in1(1,:)).*cos(in1(2,:))+in1(3,:).*in1(4,:).*cos(in1(2,:)).*sin(in1(1,:))+in1(3,:).*in1(5,:).*cos(in1(1,:)).*sin(in1(2,:)),-in1(6,:).*sin(in1(2,:))-in1(3,:).*in1(5,:).*cos(in1(2,:)),in1(4,:).*cos(in1(1,:)).*sin(in1(2,:))+in1(5,:).*cos(in1(2,:)).*sin(in1(1,:)),-in1(5,:).*cos(in1(1,:)).*cos(in1(2,:))+in1(4,:).*sin(in1(1,:)).*sin(in1(2,:)),-in1(5,:).*sin(in1(2,:))],[3,3]);
JLdot=f_JLdot([q;qdot]);
end

== matlab function RobotSimulation/Controllers/MATLAB Function1 ==
  data: t input; x output; v output; a output
function [x,v,a] = t2xyz(t)
T=2;
X0=0.1; Y0=0.05; Z0=0.25;
dX=0.15; dY=-0.2; dZ=0.1;

x=(10*(t/T)^3-15*(t/T)^4+6*(t/T)^5)*[dX,dY,dZ]'+[X0,Y0,Z0]';
v=(30*(t^2)/T^3-60*(t^3)/T^4+30*(t^4)/T^5)*[dX,dY,dZ]';
a=(60*t/T^3-180*(t^2)/T^4+120*(t^3)/T^5)*[dX,dY,dZ]';
end

== matlab function RobotSimulation/Direct Kinematics ==
  data: T output; q input
function T = fcn(q)
f_A3t0=@(in1)reshape([cos(in1(1,:)),sin(in1(1,:)),0.0,0.0,-cos(in1(2,:)).*sin(in1(1,:)),cos(in1(1,:)).*cos(in1(2,:)),sin(in1(2,:)),0.0,sin(in1(1,:)).*sin(in1(2,:)),-cos(in1(1,:)).*sin(in1(2,:)),cos(in1(2,:)),0.0,cos(in1(1,:))./1.0e+1+in1(3,:).*sin(in1(1,:)).*sin(in1(2,:)),sin(in1(1,:))./1.0e+1-in1(3,:).*cos(in1(1,:)).*sin(in1(2,:)),in1(3,:).*cos(in1(2,:))+1.0./5.0,1.0],[4,4]);
A=f_A3t0(q);
T=A(1:3,4);
end

== matlab function RobotSimulation/Initialize Function/MATLAB Function1 ==
  data: t input; x output; v output; a output
function [x,v,a] = t2xyz(t)
T=2;
X0=0.1; Y0=0.05; Z0=0.25;
dX=0.15; dY=-0.2; dZ=0.1;

x=(10*(t/T)^3-15*(t/T)^4+6*(t/T)^5)*[dX,dY,dZ]'+[X0,Y0,Z0]';
v=(30*(t^2)/T^3-60*(t^3)/T^4+30*(t^4)/T^5)*[dX,dY,dZ]';
a=(60*t/T^3-180*(t^2)/T^4+120*(t^3)/T^5)*[dX,dY,dZ]';
end

== matlab function RobotSimulation/Initialize Function/MATLAB Function ==
  data: x input; v input; a input; q output; elbows input; q_dot output; q_dot2 output
function [q,q_dot,q_dot2] = xyz2q(x,v,a,elbows)
q=inverse_kin(x,elbows);

JL=CalcJL(q);
q_dot=linsolve((JL),v);

JL_dot=CalcJLdot(q,q_dot);
q_dot2=linsolve(JL,a-JL_dot*q_dot);
end

function q=inverse_kin(x,elbows)
H=0.2;
L=0.1;

t2_elbow=elbows(1);
d3_elbow=elbows(2);
q=zeros(3,size(x,2));
for i=1:size(x,2)
    %Parse
    Px=x(1,i);
    Py=x(2,i);
    Pz=x(3,i);
    %Compute d3
    d3=d3_elbow*sqrt(Px^2+Py^2+(Pz-H)^2-L^2);
    %compute theta2
    c2=(Pz-H)/(d3+eps); %<------------Added eps
    s2=t2_elbow*sqrt(1-c2^2);
    t2=atan2(s2,c2);
    %compute theta1
    a=d3*s2;
    b=L;
    c=-Py;
    d=Px;
    t1=atan2(a*d-b*c,a*c+b*d);
    %create joint vector
    q(:,i)=[t1,t2,d3]';
end
end

function JL=CalcJL(q)
f_JL=@(in1)reshape([sin(in1(1,:)).*(-1.0./1.0e+1)+in1(3,:).*cos(in1(1,:)).*sin(in1(2,:)),cos(in1(1,:))./1.0e+1+in1(3,:).*sin(in1(1,:)).*sin(in1(2,:)),0.0,in1(3,:).*cos(in1(2,:)).*sin(in1(1,:)),-in1(3,:).*cos(in1(1,:)).*cos(in1(2,:)),-in1(3,:).*sin(in1(2,:)),sin(in1(1,:)).*sin(in1(2,:)),-cos(in1(1,:)).*sin(in1(2,:)),cos(in1(2,:))],[3,3]);
JL=f_JL(q);
end

function JLdot=CalcJLdot(q,qdot)
f_JLdot=@(in1)reshape([-in1(4,:).*(cos(in1(1,:))./1.0e+1+in1(3,:).*sin(in1(1,:)).*sin(in1(2,:)))+in1(6,:).*cos(in1(1,:)).*sin(in1(2,:))+in1(3,:).*in1(5,:).*cos(in1(1,:)).*cos(in1(2,:)),-in1(4,:).*(sin(in1(1,:))./1.0e+1-in1(3,:).*cos(in1(1,:)).*sin(in1(2,:)))+in1(6,:).*sin(in1(1,:)).*sin(in1(2,:))+in1(3,:).*in1(5,:).*cos(in1(2,:)).*sin(in1(1,:)),0.0,in1(6,:).*cos(in1(2,:)).*sin(in1(1,:))-in1(3,:).*in1(5,:).*sin(in1(1,:)).*sin(in1(2,:))+in1(3,:).*in1(4,:).*cos(in1(1,:)).*cos(in1(2,:)),-in1(6,:).*cos(in1(1,:)).*cos(in1(2,:))+in1(3,:).*in1(4,:).*cos(in1(2,:)).*sin(in1(1,:))+in1(3,:).*in1(5,:).*cos(in1(1,:)).*sin(in1(2,:)),-in1(6,:).*sin(in1(2,:))-in1(3,:).*in1(5,:).*cos(in1(2,:)),in1(4,:).*cos(in1(1,:)).*sin(in1(2,:))+in1(5,:).*cos(in1(2,:)).*sin(in1(1,:)),-in1(5,:).*cos(in1(1,:)).*cos(in1(2,:))+in1(4,:).*sin(in1(1,:)).*sin(in1(2,:)),-in1(5,:).*sin(in1(2,:))],[3,3]);
JLdot=f_JLdot([q;qdot]);
end

== matlab function RobotSimulation/Controllers/Subsystem/Compute C ==
  data: q input; C output; qdot input; Mchoice input
function C = ComputeC(q,qdot,Mchoice)
f_CdynM1=@(in1)reshape([in1(6,:).*((in1(3,:).*sin(in1(2,:)).^2)./2.0-pi.*sin(in1(2,:)).^2.*2.19375e-3+in1(3,:).*pi.*sin(in1(2,:)).^2.*4.3875e-2)+in1(5,:).*((in1(3,:).^2.*sin(in1(2,:).*2.0))./4.0+pi.*sin(in1(2,:).*2.0).*7.3125e-5-in1(3,:).*pi.*sin(in1(2,:).*2.0).*2.19375e-3+in1(3,:).^2.*pi.*sin(in1(2,:).*2.0).*2.19375e-2),in1(4,:).*sin(in1(2,:).*2.0).*(pi.*1.755e-1-in1(3,:).*pi.*5.265+in1(3,:).^2.*pi.*5.265e+1+in1(3,:).^2.*6.0e+2).*(-4.166666666666667e-4),in1(4,:).*sin(in1(2,:)).^2.*(in1(3,:).*1.0e+1-pi.*4.3875e-2+in1(3,:).*pi.*(3.51e+2./4.0e+2)).*(-1.0./2.0e+1),in1(4,:).*((in1(3,:).^2.*sin(in1(2,:).*2.0))./4.0+pi.*sin(in1(2,:).*2.0).*7.3125e-5-in1(3,:).*pi.*sin(in1(2,:).*2.0).*2.19375e-3+in1(3,:).^2.*pi.*sin(in1(2,:).*2.0).*2.19375e-2)-in1(6,:).*((cos(in1(2,:)).*(pi.*(3.51e+2./4.0e+2)+1.0e+1))./4.0e+2+(cos(in1(2,:)).*(pi.*4.3875e-2+1.0./2.0))./2.0e+1)+(in1(5,:).*sin(in1(2,:)).*(in1(3,:).*1.0e+1-pi.*4.3875e-2+in1(3,:).*pi.*(3.51e+2./4.0e+2)))./2.0e+2,in1(6,:).*(in1(3,:)./2.0+pi.*(in1(3,:).*2.0-1.0./1.0e+1).*2.19375e-2),in1(5,:).*(in1(3,:).*1.0e+1-pi.*4.3875e-2+in1(3,:).*pi.*(3.51e+2./4.0e+2)).*(-1.0./2.0e+1),-in1(4,:).*(pi.*(cos(in1(2,:)).^2-1.0).*(-2.19375e-3)+(in1(3,:).*(cos(in1(2,:)).^2-1.0))./2.0+in1(3,:).*pi.*(cos(in1(2,:)).^2-1.0).*4.3875e-2)-in1(5,:).*((cos(in1(2,:)).*(pi.*(3.51e+2./4.0e+2)+1.0e+1))./4.0e+2+(cos(in1(2,:)).*(pi.*4.3875e-2+1.0./2.0))./2.0e+1),(in1(5,:).*(in1(3,:).*1.0e+1-pi.*4.3875e-2+in1(3,:).*pi.*(3.51e+2./4.0e+2)))./2.0e+1,0.0],[3,3]);
f_CdynM2=@(in1)reshape([in1(6,:).*(in1(3,:).*sin(in1(2,:)).^2.*(3.0./5.0)-pi.*sin(in1(2,:)).^2.*2.19375e-3+in1(3,:).*pi.*sin(in1(2,:)).^2.*4.3875e-2)+in1(5,:).*(in1(3,:).^2.*sin(in1(2,:).*2.0).*(3.0./1.0e+1)+pi.*sin(in1(2,:).*2.0).*7.3125e-5-in1(3,:).*pi.*sin(in1(2,:).*2.0).*2.19375e-3+in1(3,:).^2.*pi.*sin(in1(2,:).*2.0).*2.19375e-2),in1(4,:).*sin(in1(2,:).*2.0).*(pi.*1.755e-1-in1(3,:).*pi.*5.265+in1(3,:).^2.*pi.*5.265e+1+in1(3,:).^2.*7.2e+2).*(-4.166666666666667e-4),in1(4,:).*sin(in1(2,:)).^2.*(in1(3,:).*1.2e+1-pi.*4.3875e-2+in1(3,:).*pi.*(3.51e+2./4.0e+2)).*(-1.0./2.0e+1),in1(4,:).*(in1(3,:).^2.*sin(in1(2,:).*2.0).*(3.0./1.0e+1)+pi.*sin(in1(2,:).*2.0).*7.3125e-5-in1(3,:).*pi.*sin(in1(2,:).*2.0).*2.19375e-3+in1(3,:).^2.*pi.*sin(in1(2,:).*2.0).*2.19375e-2)-in1(6,:).*((cos(in1(2,:)).*(pi.*(3.51e+2./4.0e+2)+1.2e+1))./4.0e+2+(cos(in1(2,:)).*(pi.*4.3875e-2+3.0./5.0))./2.0e+1)+(in1(5,:).*sin(in1(2,:)).*(in1(3,:).*1.2e+1-pi.*4.3875e-2+in1(3,:).*pi.*(3.51e+2./4.0e+2)))./2.0e+2,in1(6,:).*(in1(3,:).*(3.0./5.0)+pi.*(in1(3,:).*2.0-1.0./1.0e+1).*2.19375e-2),in1(5,:).*(in1(3,:).*1.2e+1-pi.*4.3875e-2+in1(3,:).*pi.*(3.51e+2./4.0e+2)).*(-1.0./2.0e+1),-in1(4,:).*(pi.*(cos(in1(2,:)).^2-1.0).*(-2.19375e-3)+in1(3,:).*(cos(in1(2,:)).^2-1.0).*(3.0./5.0)+in1(3,:).*pi.*(cos(in1(2,:)).^2-1.0).*4.3875e-2)-in1(5,:).*((cos(in1(2,:)).*(pi.*(3.51e+2./4.0e+2)+1.2e+1))./4.0e+2+(cos(in1(2,:)).*(pi.*4.3875e-2+3.0./5.0))./2.0e+1),(in1(5,:).*(in1(3,:).*1.2e+1-pi.*4.3875e-2+in1(3,:).*pi.*(3.51e+2./4.0e+2)))./2.0e+1,0.0],[3,3]);
if Mchoice==1
    C=f_CdynM1([q;qdot]);
else %==2
    C=f_CdynM2([q;qdot]);
end
end
